simulink model "ex7_1"  (R2020a)
settings: Solver=VariableStepAuto  StartTime=0.0  StopTime=10.0  RelTol=1e-3
settings Model: Creator=반달  LastModifiedBy=반달
settings DataIOCC: ReturnWorkspaceOutputs=off

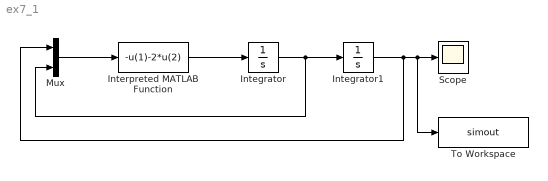
== system ex7_1 ==
  Integrator : Integrator
  Integrator1 : Integrator  InitialCondition=2
  Interpreted MATLAB Function : MATLABFcn  MATLABFcn=-u(1)-2*u(2)
  Mux : Mux  Inputs=2
  Scope : Scope
  To Workspace : ToWorkspace  VariableName=simout  SaveFormat=Structure With Time  SampleTime=-1
  wires:
  Interpreted MATLAB Function/1 -> Integrator/1
  Mux/1 -> Interpreted MATLAB Function/1
  Integrator/1 -> Mux/2, Integrator1/1
  Integrator1/1 -> Mux/1, To Workspace/1, Scope/1
